simulink model "NCOtest"  (Simulink 7.9)
settings: Solver=ode45  StartTime=0.0  StopTime=.1  RelTol=1e-3
values from neighbouring files (symbols this model uses):
  D = [  1 -1  1 -1  1  1 -1 -1 ... (first row only)    [cdma.m]    (also in compressed_sampling.m = idct(eye(5000,5000)))
undefined symbols (not defined in the file or in its folder): Fsymbol
libraries: dspsigops x2
settings Model: Creator=ArunKB  LastModifiedBy=ArunKB

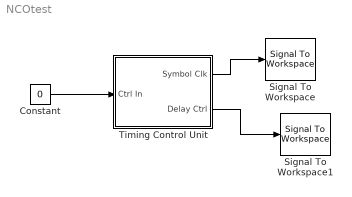
== system NCOtest ==
  Constant : Constant  Value=0  OutDataTypeStr=Inherit: Inherit via back propagation  SampleTime=1/(Fsymbol*D/2)
  Signal To Workspace : SignalToWorkspace  VariableName=yout
      settings: CopyFcn=dspblkcopystw(gcbh);
  Signal To Workspace1 : SignalToWorkspace  VariableName=yout1
      settings: CopyFcn=dspblkcopystw(gcbh);
  Timing Control Unit : Subsystem
  wires:
  Constant/1 -> Timing Control Unit/1(Ctrl In)
  Timing Control Unit/1(Symbol Clk) -> Signal To Workspace/1
  Timing Control Unit/2(Delay Ctrl) -> Signal To Workspace1/1

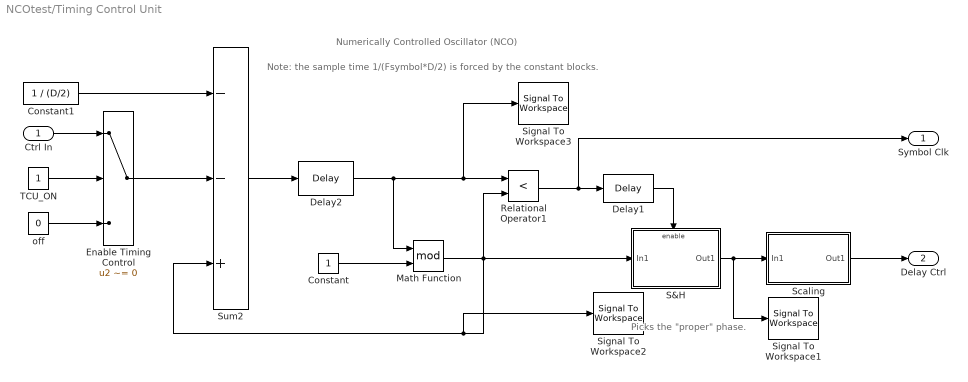
== system NCOtest/Timing Control Unit ==
  note: Picks the "proper" phase.
  note: Numerically Controlled Oscillator (NCO)
  note: Note:  the sample time 1/(Fsymbol*D/2)
      | is forced by the constant blocks.
  Ctrl In : Inport
  Constant : Constant  OutDataTypeStr=Inherit: Inherit via back propagation  SampleTime=1/(Fsymbol*D/2)
  Constant1 : Constant  Value=1 / (D/2)  OutDataTypeStr=Inherit: Inherit via back propagation  SampleTime=1/(Fsymbol*D/2)
  Delay1 : dspsigops/Delay  dly_unit=Samples  delay=1  ic_detail=off  dif_ic_for_ch=off  dif_ic_for_dly=off  ic=0  reset_popup=None
  Delay2 : dspsigops/Delay  dly_unit=Samples  delay=1  ic_detail=on  dif_ic_for_ch=off  dif_ic_for_dly=off  ic=0  reset_popup=None
  Enable Timing Control : Switch  Criteria=u2 ~= 0
  Math Function : Math  Operator=mod  SaturateOnIntegerOverflow=on
  Relational Operator1 : RelationalOperator  Operator=<  OutDataTypeStr=boolean
  "S&H " : Subsystem  TreatAsAtomicUnit=on
  Scaling : Subsystem
  Signal To Workspace1 : SignalToWorkspace  VariableName=yout3
      settings: CopyFcn=dspblkcopystw(gcbh);
  Signal To Workspace2 : SignalToWorkspace  VariableName=yout2
      settings: CopyFcn=dspblkcopystw(gcbh);
  Signal To Workspace3 : SignalToWorkspace  VariableName=yout4
      settings: CopyFcn=dspblkcopystw(gcbh);
  Sum2 : Sum  Inputs=--+  SaturateOnIntegerOverflow=on  InputSameDT=on  OutDataTypeStr=Inherit: Same as first input
  TCU_ON : Constant  OutDataTypeStr=boolean
  off : Constant  Value=0
  Symbol Clk : Outport
  Delay Ctrl : Outport  Port=2
  wires:
  Enable Timing Control/1 -> Sum2/2
  Ctrl In/1 -> Enable Timing Control/1
  off/1 -> Enable Timing Control/3
  TCU_ON/1 -> Enable Timing Control/2
  Scaling/1(Out1) -> Delay Ctrl/1
  "S&H "/1(Out1) -> Scaling/1(In1), Signal To Workspace1/1
  Delay1/1 -> "S&H "/Enable
  Relational Operator1/1 -> Symbol Clk/1, Delay1/1
  Math Function/1 -> "S&H "/1(In1), Relational Operator1/2, Sum2/3, Signal To Workspace2/1
  Constant1/1 -> Sum2/1
  Sum2/1 -> Delay2/1
  Constant/1 -> Math Function/2
  Delay2/1 -> Math Function/1, Relational Operator1/1, Signal To Workspace3/1

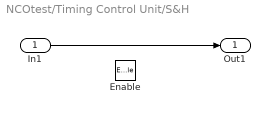
== system NCOtest/Timing Control Unit/S&H  ==
  In1 : Inport
  Enable : EnablePort  PropagateVarSize=During execution
  Out1 : Outport
  wires:
  In1/1 -> Out1/1

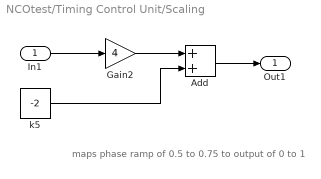
== system NCOtest/Timing Control Unit/Scaling ==
  note: maps phase ramp of 0.5 to 0.75 to output of 0 to 1
  In1 : Inport
  Add : Sum
  Gain2 : Gain  Gain=4
  k5 : Constant  Value=-2  SampleTime=1/(Fsymbol*D/2)
  Out1 : Outport
  wires:
  Gain2/1 -> Add/1
  k5/1 -> Add/2
  In1/1 -> Gain2/1
  Add/1 -> Out1/1
